simulink library "lib_outputs"  (Simulink 4.1.1)
undefined symbols (not defined in the file or in its folder): ess2_init_soc, ess_init_soc
libraries: lib_outputs x2
settings Model: LastModifiedBy=abrooker  ModifiedComment=abrooker -- Thu Apr 25 12:43:46 2002 -- Version 1.75
settings Model: ModifiedHistory=|
  | abrooker -- Thu Apr 25 12:43:46 2002 -- Version 1.75
  | 
  | 
  | abrooker -- Thu Apr 25 12:43:39 2002 -- Version 1.74
  | 
  | 
  | abrooker -- Thu Apr 25 12:37:48 2002 -- Version 1.73
  | 
  | 
  | abrooker -- Thu Apr 25 11:19:32 2002 -- Version 1.72
  | 
  | 
  | abrooker -- Thu Apr 25 11:09:29 2002 -- Version 1.71
  | 
  | 
  | abrooker -- Thu Apr 25 11:09:22 2002 -- Version 1.70
  | 
  | 
  | mokeefe -- Thu Apr 18 08:37:41 2002 -- Version 1.69
  | saving the model:
  | o "without the model browser open"
  | o with only top-level screen visible
  | o with "fit to view" enabled
  | o with "status bar" off and "toolbar" off
  | o with "prompt to update model history with each save" on

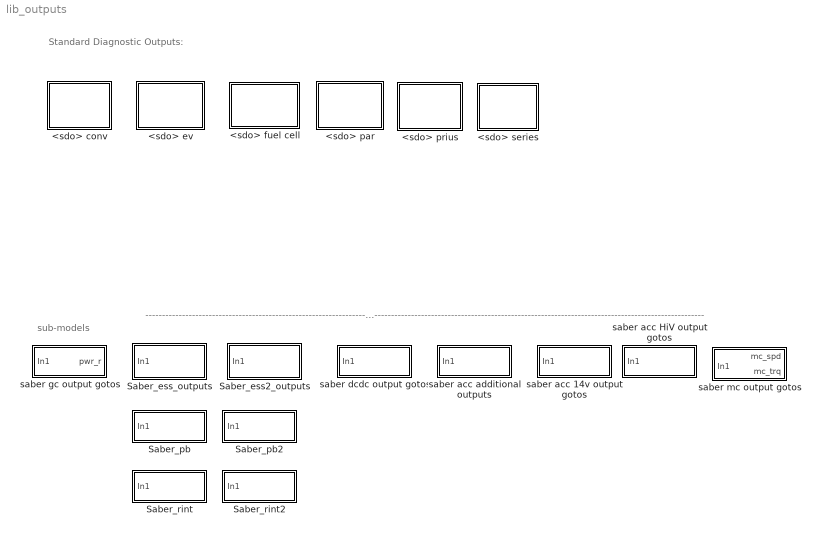
== system lib_outputs ==
  note: Standard Diagnostic Outputs:
  note: sub-models
  note: ------------------------------------------------------------------------------------------------------------------------------------------------------------------------------------------------------------------
  <sdo> conv : Subsystem
      settings: RTWFcnNameOpts=Auto  RTWFileNameOpts=Auto
      mask Display: image(imread('bdi_sdo.jpg'))
  <sdo> ev : Subsystem
      settings: RTWFcnNameOpts=Auto  RTWFileNameOpts=Auto
      mask Display: image(imread('bdi_sdo.jpg'))
  <sdo> fuel cell : Subsystem
      settings: RTWFcnNameOpts=Auto  RTWFileNameOpts=Auto
      mask Display: image(imread('bdi_sdo.jpg'))
  <sdo> par : Subsystem
      settings: RTWFcnNameOpts=Auto  RTWFileNameOpts=Auto
      mask Display: image(imread('bdi_sdo.jpg'))
  <sdo> prius : Subsystem
      settings: RTWFcnNameOpts=Auto  RTWFileNameOpts=Auto
      mask Display: image(imread('bdi_sdo.jpg'))
  <sdo> series : Subsystem
      settings: RTWFcnNameOpts=Auto  RTWFileNameOpts=Auto
      mask Display: image(imread('bdi_sdo.jpg'))
  Saber_ess2_outputs : Subsystem  BlockChoice=Saber_rint2
      settings: TemplateBlock=self  MemberBlocks=Saber_pb2,Saber_rint2  RTWFcnNameOpts=Auto  RTWFileNameOpts=Auto
  Saber_ess_outputs : Subsystem  BlockChoice=Saber_rint
      settings: TemplateBlock=self  MemberBlocks=Saber_pb,Saber_rint  RTWFcnNameOpts=Auto  RTWFileNameOpts=Auto
  Saber_pb : Subsystem
      settings: RTWFcnNameOpts=Auto  RTWFileNameOpts=Auto
  Saber_pb2 : Subsystem
      settings: RTWFcnNameOpts=Auto  RTWFileNameOpts=Auto
  Saber_rint : Subsystem
      settings: RTWFcnNameOpts=Auto  RTWFileNameOpts=Auto
  Saber_rint2 : Subsystem
      settings: RTWFcnNameOpts=Auto  RTWFileNameOpts=Auto
  saber acc 14v output gotos : Subsystem
      settings: RTWFcnNameOpts=Auto  RTWFileNameOpts=Auto
  saber acc HiV output gotos : Subsystem
      settings: RTWFcnNameOpts=Auto  RTWFileNameOpts=Auto
  saber acc additional outputs : Subsystem
      settings: RTWFcnNameOpts=Auto  RTWFileNameOpts=Auto
  saber dcdc output gotos : Subsystem
      settings: RTWFcnNameOpts=Auto  RTWFileNameOpts=Auto
  saber gc output gotos : Subsystem
      settings: RTWFcnNameOpts=Auto  RTWFileNameOpts=Auto
  saber mc output gotos : Subsystem
      settings: RTWFcnNameOpts=Auto  RTWFileNameOpts=Auto

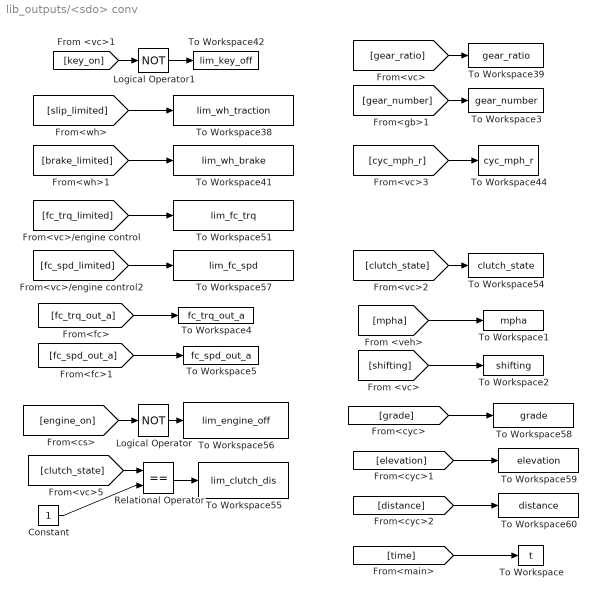
== system lib_outputs/<sdo> conv ==
  Constant : Constant  Value=1
  Logical Operator : Logic  Operator=NOT  Inputs=1
  Logical Operator1 : Logic  Operator=NOT  Inputs=1
  Relational Operator : RelationalOperator  Operator===
  To Workspace : ToWorkspace  VariableName=t  SampleTime=0  SaveFormat=Array
  To Workspace1 : ToWorkspace  VariableName=mpha  SampleTime=-1  SaveFormat=Array
  To Workspace2 : ToWorkspace  VariableName=shifting  SampleTime=-1  SaveFormat=Array
  To Workspace3 : ToWorkspace  VariableName=gear_number  SampleTime=-1  SaveFormat=Array
  To Workspace38 : ToWorkspace  VariableName=lim_wh_traction  SampleTime=-1  SaveFormat=Array
  To Workspace39 : ToWorkspace  VariableName=gear_ratio  SampleTime=-1  SaveFormat=Array
  To Workspace4 : ToWorkspace  VariableName=fc_trq_out_a  SampleTime=-1  SaveFormat=Array
  To Workspace41 : ToWorkspace  VariableName=lim_wh_brake  SampleTime=-1  SaveFormat=Array
  To Workspace42 : ToWorkspace  VariableName=lim_key_off  SampleTime=-1  SaveFormat=Array
  To Workspace44 : ToWorkspace  VariableName=cyc_mph_r  SampleTime=-1  SaveFormat=Array
  To Workspace5 : ToWorkspace  VariableName=fc_spd_out_a  SampleTime=-1  SaveFormat=Array
  To Workspace51 : ToWorkspace  VariableName=lim_fc_trq  SampleTime=-1  SaveFormat=Array
  To Workspace54 : ToWorkspace  VariableName=clutch_state  SampleTime=-1  SaveFormat=Array
  To Workspace55 : ToWorkspace  VariableName=lim_clutch_dis  SampleTime=-1  SaveFormat=Array
  To Workspace56 : ToWorkspace  VariableName=lim_engine_off  SampleTime=-1  SaveFormat=Array
  To Workspace57 : ToWorkspace  VariableName=lim_fc_spd  SampleTime=-1  SaveFormat=Array
  To Workspace58 : ToWorkspace  VariableName=grade  SampleTime=-1  SaveFormat=Array
  To Workspace59 : ToWorkspace  VariableName=elevation  SampleTime=-1  SaveFormat=Array
  To Workspace60 : ToWorkspace  VariableName=distance  SampleTime=-1  SaveFormat=Array
  wires:
  [gear_ratio] -> To Workspace39/1
  [cyc_mph_r] -> To Workspace44/1
  [clutch_state] -> To Workspace54/1
  [mpha] -> To Workspace1/1
  [shifting] -> To Workspace2/1
  [slip_limited] -> To Workspace38/1
  [brake_limited] -> To Workspace41/1
  [fc_trq_limited] -> To Workspace51/1
  [fc_spd_limited] -> To Workspace57/1
  [key_on] -> Logical Operator1/1
  Logical Operator1/1 -> To Workspace42/1
  [grade] -> To Workspace58/1
  [elevation] -> To Workspace59/1
  [distance] -> To Workspace60/1
  [clutch_state] -> Relational Operator/1
  Relational Operator/1 -> To Workspace55/1
  Constant/1 -> Relational Operator/2
  [engine_on] -> Logical Operator/1
  Logical Operator/1 -> To Workspace56/1
  [fc_trq_out_a] -> To Workspace4/1
  [fc_spd_out_a] -> To Workspace5/1
  [time] -> To Workspace/1
  [gear_number] -> To Workspace3/1

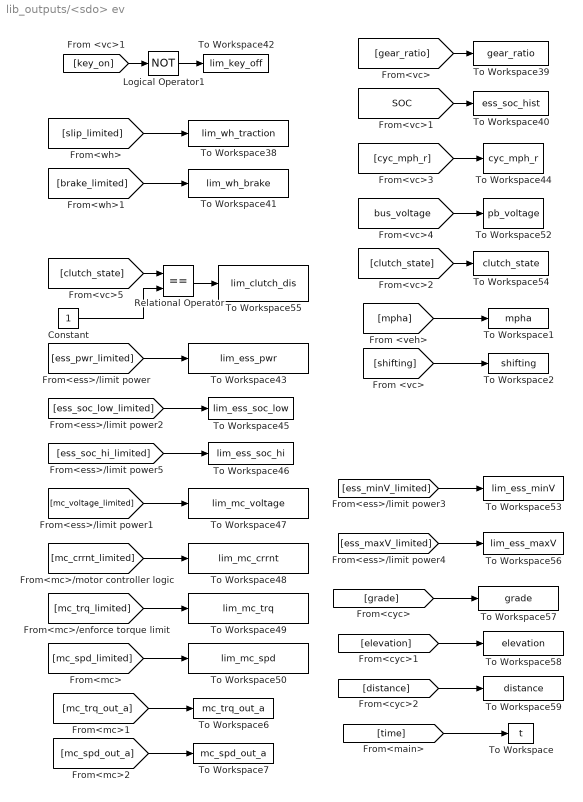
== system lib_outputs/<sdo> ev ==
  Constant : Constant  Value=1
  Logical Operator1 : Logic  Operator=NOT  Inputs=1
  Relational Operator : RelationalOperator  Operator===
  To Workspace : ToWorkspace  VariableName=t  SampleTime=0  SaveFormat=Array
  To Workspace1 : ToWorkspace  VariableName=mpha  SampleTime=-1  SaveFormat=Array
  To Workspace2 : ToWorkspace  VariableName=shifting  SampleTime=-1  SaveFormat=Array
  To Workspace38 : ToWorkspace  VariableName=lim_wh_traction  SampleTime=-1  SaveFormat=Array
  To Workspace39 : ToWorkspace  VariableName=gear_ratio  SampleTime=-1  SaveFormat=Array
  To Workspace40 : ToWorkspace  VariableName=ess_soc_hist  SampleTime=-1  SaveFormat=Array
  To Workspace41 : ToWorkspace  VariableName=lim_wh_brake  SampleTime=-1  SaveFormat=Array
  To Workspace42 : ToWorkspace  VariableName=lim_key_off  SampleTime=-1  SaveFormat=Array
  To Workspace43 : ToWorkspace  VariableName=lim_ess_pwr  SampleTime=-1  SaveFormat=Array
  To Workspace44 : ToWorkspace  VariableName=cyc_mph_r  SampleTime=-1  SaveFormat=Array
  To Workspace45 : ToWorkspace  VariableName=lim_ess_soc_low  SampleTime=-1  SaveFormat=Array
  To Workspace46 : ToWorkspace  VariableName=lim_ess_soc_hi  SampleTime=-1  SaveFormat=Array
  To Workspace47 : ToWorkspace  VariableName=lim_mc_voltage  SampleTime=-1  SaveFormat=Array
  To Workspace48 : ToWorkspace  VariableName=lim_mc_crrnt  SampleTime=-1  SaveFormat=Array
  To Workspace49 : ToWorkspace  VariableName=lim_mc_trq  SampleTime=-1  SaveFormat=Array
  To Workspace50 : ToWorkspace  VariableName=lim_mc_spd  SampleTime=-1  SaveFormat=Array
  To Workspace52 : ToWorkspace  VariableName=pb_voltage  SampleTime=-1  SaveFormat=Array
  To Workspace53 : ToWorkspace  VariableName=lim_ess_minV  SampleTime=-1  SaveFormat=Array
  To Workspace54 : ToWorkspace  VariableName=clutch_state  SampleTime=-1  SaveFormat=Array
  To Workspace55 : ToWorkspace  VariableName=lim_clutch_dis  SampleTime=-1  SaveFormat=Array
  To Workspace56 : ToWorkspace  VariableName=lim_ess_maxV  SampleTime=-1  SaveFormat=Array
  To Workspace57 : ToWorkspace  VariableName=grade  SampleTime=-1  SaveFormat=Array
  To Workspace58 : ToWorkspace  VariableName=elevation  SampleTime=-1  SaveFormat=Array
  To Workspace59 : ToWorkspace  VariableName=distance  SampleTime=-1  SaveFormat=Array
  To Workspace6 : ToWorkspace  VariableName=mc_trq_out_a  SampleTime=-1  SaveFormat=Array
  To Workspace7 : ToWorkspace  VariableName=mc_spd_out_a  SampleTime=-1  SaveFormat=Array
  wires:
  [mc_voltage_limited] -> To Workspace47/1
  [mc_crrnt_limited] -> To Workspace48/1
  [mc_trq_limited] -> To Workspace49/1
  [mc_spd_limited] -> To Workspace50/1
  [gear_ratio] -> To Workspace39/1
  [cyc_mph_r] -> To Workspace44/1
  [SOC] -> To Workspace40/1
  [bus_voltage] -> To Workspace52/1
  [clutch_state] -> To Workspace54/1
  [mpha] -> To Workspace1/1
  [shifting] -> To Workspace2/1
  [slip_limited] -> To Workspace38/1
  [brake_limited] -> To Workspace41/1
  [key_on] -> Logical Operator1/1
  Logical Operator1/1 -> To Workspace42/1
  [ess_maxV_limited] -> To Workspace56/1
  [ess_minV_limited] -> To Workspace53/1
  [grade] -> To Workspace57/1
  [elevation] -> To Workspace58/1
  [distance] -> To Workspace59/1
  [ess_pwr_limited] -> To Workspace43/1
  [clutch_state] -> Relational Operator/1
  Relational Operator/1 -> To Workspace55/1
  Constant/1 -> Relational Operator/2
  [ess_soc_low_limited] -> To Workspace45/1
  [ess_soc_hi_limited] -> To Workspace46/1
  [time] -> To Workspace/1
  [mc_trq_out_a] -> To Workspace6/1
  [mc_spd_out_a] -> To Workspace7/1

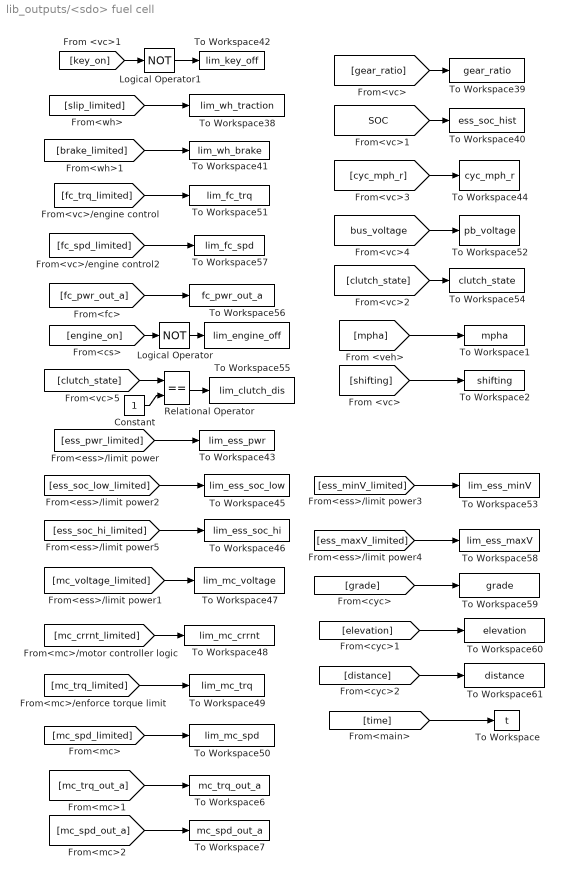
== system lib_outputs/<sdo> fuel cell ==
  " " : ToWorkspace  VariableName=fc_pwr_out_a  SampleTime=-1  SaveFormat=Array
  Constant : Constant  Value=1
  Logical Operator : Logic  Operator=NOT  Inputs=1
  Logical Operator1 : Logic  Operator=NOT  Inputs=1
  Relational Operator : RelationalOperator  Operator===
  To Workspace : ToWorkspace  VariableName=t  SampleTime=0  SaveFormat=Array
  To Workspace1 : ToWorkspace  VariableName=mpha  SampleTime=-1  SaveFormat=Array
  To Workspace2 : ToWorkspace  VariableName=shifting  SampleTime=-1  SaveFormat=Array
  To Workspace38 : ToWorkspace  VariableName=lim_wh_traction  SampleTime=-1  SaveFormat=Array
  To Workspace39 : ToWorkspace  VariableName=gear_ratio  SampleTime=-1  SaveFormat=Array
  To Workspace40 : ToWorkspace  VariableName=ess_soc_hist  SampleTime=-1  SaveFormat=Array
  To Workspace41 : ToWorkspace  VariableName=lim_wh_brake  SampleTime=-1  SaveFormat=Array
  To Workspace42 : ToWorkspace  VariableName=lim_key_off  SampleTime=-1  SaveFormat=Array
  To Workspace43 : ToWorkspace  VariableName=lim_ess_pwr  SampleTime=-1  SaveFormat=Array
  To Workspace44 : ToWorkspace  VariableName=cyc_mph_r  SampleTime=-1  SaveFormat=Array
  To Workspace45 : ToWorkspace  VariableName=lim_ess_soc_low  SampleTime=-1  SaveFormat=Array
  To Workspace46 : ToWorkspace  VariableName=lim_ess_soc_hi  SampleTime=-1  SaveFormat=Array
  To Workspace47 : ToWorkspace  VariableName=lim_mc_voltage  SampleTime=-1  SaveFormat=Array
  To Workspace48 : ToWorkspace  VariableName=lim_mc_crrnt  SampleTime=-1  SaveFormat=Array
  To Workspace49 : ToWorkspace  VariableName=lim_mc_trq  SampleTime=-1  SaveFormat=Array
  To Workspace50 : ToWorkspace  VariableName=lim_mc_spd  SampleTime=-1  SaveFormat=Array
  To Workspace51 : ToWorkspace  VariableName=lim_fc_trq  SampleTime=-1  SaveFormat=Array
  To Workspace52 : ToWorkspace  VariableName=pb_voltage  SampleTime=-1  SaveFormat=Array
  To Workspace53 : ToWorkspace  VariableName=lim_ess_minV  SampleTime=-1  SaveFormat=Array
  To Workspace54 : ToWorkspace  VariableName=clutch_state  SampleTime=-1  SaveFormat=Array
  To Workspace55 : ToWorkspace  VariableName=lim_clutch_dis  SampleTime=-1  SaveFormat=Array
  To Workspace56 : ToWorkspace  VariableName=lim_engine_off  SampleTime=-1  SaveFormat=Array
  To Workspace57 : ToWorkspace  VariableName=lim_fc_spd  SampleTime=-1  SaveFormat=Array
  To Workspace58 : ToWorkspace  VariableName=lim_ess_maxV  SampleTime=-1  SaveFormat=Array
  To Workspace59 : ToWorkspace  VariableName=grade  SampleTime=-1  SaveFormat=Array
  To Workspace6 : ToWorkspace  VariableName=mc_trq_out_a  SampleTime=-1  SaveFormat=Array
  To Workspace60 : ToWorkspace  VariableName=elevation  SampleTime=-1  SaveFormat=Array
  To Workspace61 : ToWorkspace  VariableName=distance  SampleTime=-1  SaveFormat=Array
  To Workspace7 : ToWorkspace  VariableName=mc_spd_out_a  SampleTime=-1  SaveFormat=Array
  wires:
  [fc_trq_limited] -> To Workspace51/1
  [fc_spd_limited] -> To Workspace57/1
  [brake_limited] -> To Workspace41/1
  [slip_limited] -> To Workspace38/1
  [gear_ratio] -> To Workspace39/1
  [cyc_mph_r] -> To Workspace44/1
  [SOC] -> To Workspace40/1
  [bus_voltage] -> To Workspace52/1
  [clutch_state] -> To Workspace54/1
  [mpha] -> To Workspace1/1
  [shifting] -> To Workspace2/1
  [key_on] -> Logical Operator1/1
  Logical Operator1/1 -> To Workspace42/1
  [ess_maxV_limited] -> To Workspace58/1
  [ess_minV_limited] -> To Workspace53/1
  [grade] -> To Workspace59/1
  [elevation] -> To Workspace60/1
  [distance] -> To Workspace61/1
  [clutch_state] -> Relational Operator/1
  Relational Operator/1 -> To Workspace55/1
  Constant/1 -> Relational Operator/2
  [engine_on] -> Logical Operator/1
  Logical Operator/1 -> To Workspace56/1
  [ess_pwr_limited] -> To Workspace43/1
  [mc_voltage_limited] -> To Workspace47/1
  [mc_crrnt_limited] -> To Workspace48/1
  [mc_trq_limited] -> To Workspace49/1
  [mc_spd_limited] -> To Workspace50/1
  [ess_soc_low_limited] -> To Workspace45/1
  [ess_soc_hi_limited] -> To Workspace46/1
  [fc_pwr_out_a] -> " "/1
  [time] -> To Workspace/1
  [mc_trq_out_a] -> To Workspace6/1
  [mc_spd_out_a] -> To Workspace7/1

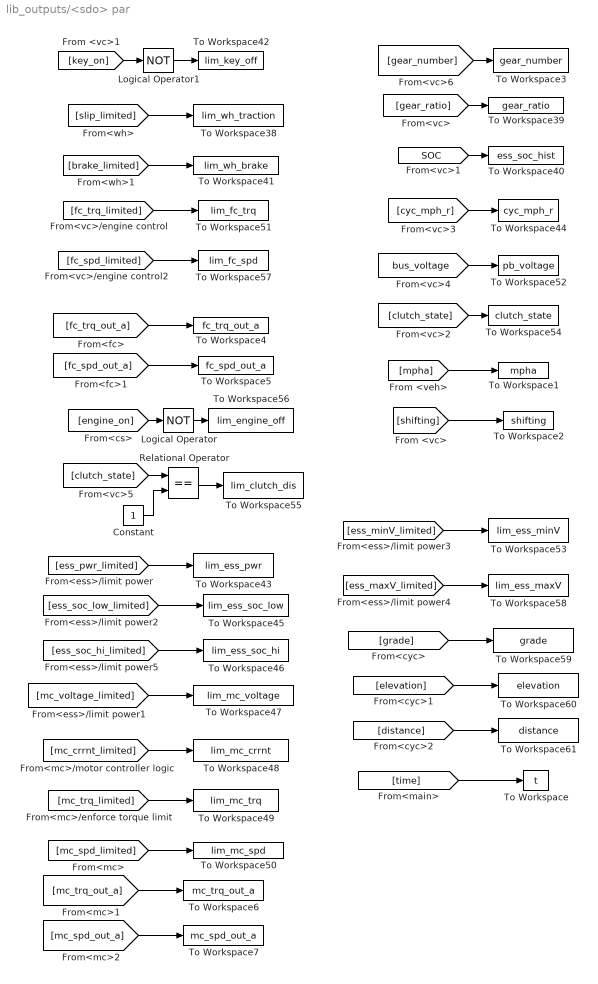
== system lib_outputs/<sdo> par ==
  Constant : Constant  Value=1
  Logical Operator : Logic  Operator=NOT  Inputs=1
  Logical Operator1 : Logic  Operator=NOT  Inputs=1
  Relational Operator : RelationalOperator  Operator===
  To Workspace : ToWorkspace  VariableName=t  SampleTime=0  SaveFormat=Array
  To Workspace1 : ToWorkspace  VariableName=mpha  SampleTime=-1  SaveFormat=Array
  To Workspace2 : ToWorkspace  VariableName=shifting  SampleTime=-1  SaveFormat=Array
  To Workspace3 : ToWorkspace  VariableName=gear_number  SampleTime=-1  SaveFormat=Array
  To Workspace38 : ToWorkspace  VariableName=lim_wh_traction  SampleTime=-1  SaveFormat=Array
  To Workspace39 : ToWorkspace  VariableName=gear_ratio  SampleTime=-1  SaveFormat=Array
  To Workspace4 : ToWorkspace  VariableName=fc_trq_out_a  SampleTime=-1  SaveFormat=Array
  To Workspace40 : ToWorkspace  VariableName=ess_soc_hist  SampleTime=-1  SaveFormat=Array
  To Workspace41 : ToWorkspace  VariableName=lim_wh_brake  SampleTime=-1  SaveFormat=Array
  To Workspace42 : ToWorkspace  VariableName=lim_key_off  SampleTime=-1  SaveFormat=Array
  To Workspace43 : ToWorkspace  VariableName=lim_ess_pwr  SampleTime=-1  SaveFormat=Array
  To Workspace44 : ToWorkspace  VariableName=cyc_mph_r  SampleTime=-1  SaveFormat=Array
  To Workspace45 : ToWorkspace  VariableName=lim_ess_soc_low  SampleTime=-1  SaveFormat=Array
  To Workspace46 : ToWorkspace  VariableName=lim_ess_soc_hi  SampleTime=-1  SaveFormat=Array
  To Workspace47 : ToWorkspace  VariableName=lim_mc_voltage  SampleTime=-1  SaveFormat=Array
  To Workspace48 : ToWorkspace  VariableName=lim_mc_crrnt  SampleTime=-1  SaveFormat=Array
  To Workspace49 : ToWorkspace  VariableName=lim_mc_trq  SampleTime=-1  SaveFormat=Array
  To Workspace5 : ToWorkspace  VariableName=fc_spd_out_a  SampleTime=-1  SaveFormat=Array
  To Workspace50 : ToWorkspace  VariableName=lim_mc_spd  SampleTime=-1  SaveFormat=Array
  To Workspace51 : ToWorkspace  VariableName=lim_fc_trq  SampleTime=-1  SaveFormat=Array
  To Workspace52 : ToWorkspace  VariableName=pb_voltage  SampleTime=-1  SaveFormat=Array
  To Workspace53 : ToWorkspace  VariableName=lim_ess_minV  SampleTime=-1  SaveFormat=Array
  To Workspace54 : ToWorkspace  VariableName=clutch_state  SampleTime=-1  SaveFormat=Array
  To Workspace55 : ToWorkspace  VariableName=lim_clutch_dis  SampleTime=-1  SaveFormat=Array
  To Workspace56 : ToWorkspace  VariableName=lim_engine_off  SampleTime=-1  SaveFormat=Array
  To Workspace57 : ToWorkspace  VariableName=lim_fc_spd  SampleTime=-1  SaveFormat=Array
  To Workspace58 : ToWorkspace  VariableName=lim_ess_maxV  SampleTime=-1  SaveFormat=Array
  To Workspace59 : ToWorkspace  VariableName=grade  SampleTime=-1  SaveFormat=Array
  To Workspace6 : ToWorkspace  VariableName=mc_trq_out_a  SampleTime=-1  SaveFormat=Array
  To Workspace60 : ToWorkspace  VariableName=elevation  SampleTime=-1  SaveFormat=Array
  To Workspace61 : ToWorkspace  VariableName=distance  SampleTime=-1  SaveFormat=Array
  To Workspace7 : ToWorkspace  VariableName=mc_spd_out_a  SampleTime=-1  SaveFormat=Array
  wires:
  [fc_trq_limited] -> To Workspace51/1
  [fc_spd_limited] -> To Workspace57/1
  [gear_ratio] -> To Workspace39/1
  [cyc_mph_r] -> To Workspace44/1
  [SOC] -> To Workspace40/1
  [bus_voltage] -> To Workspace52/1
  [clutch_state] -> To Workspace54/1
  [mpha] -> To Workspace1/1
  [shifting] -> To Workspace2/1
  [key_on] -> Logical Operator1/1
  Logical Operator1/1 -> To Workspace42/1
  [slip_limited] -> To Workspace38/1
  [brake_limited] -> To Workspace41/1
  [ess_maxV_limited] -> To Workspace58/1
  [ess_minV_limited] -> To Workspace53/1
  [grade] -> To Workspace59/1
  [elevation] -> To Workspace60/1
  [distance] -> To Workspace61/1
  [ess_pwr_limited] -> To Workspace43/1
  [clutch_state] -> Relational Operator/1
  Constant/1 -> Relational Operator/2
  [engine_on] -> Logical Operator/1
  Logical Operator/1 -> To Workspace56/1
  [ess_soc_low_limited] -> To Workspace45/1
  [ess_soc_hi_limited] -> To Workspace46/1
  [mc_voltage_limited] -> To Workspace47/1
  [mc_crrnt_limited] -> To Workspace48/1
  [mc_trq_limited] -> To Workspace49/1
  [mc_spd_limited] -> To Workspace50/1
  Relational Operator/1 -> To Workspace55/1
  [fc_trq_out_a] -> To Workspace4/1
  [fc_spd_out_a] -> To Workspace5/1
  [time] -> To Workspace/1
  [mc_trq_out_a] -> To Workspace6/1
  [mc_spd_out_a] -> To Workspace7/1
  [gear_number] -> To Workspace3/1

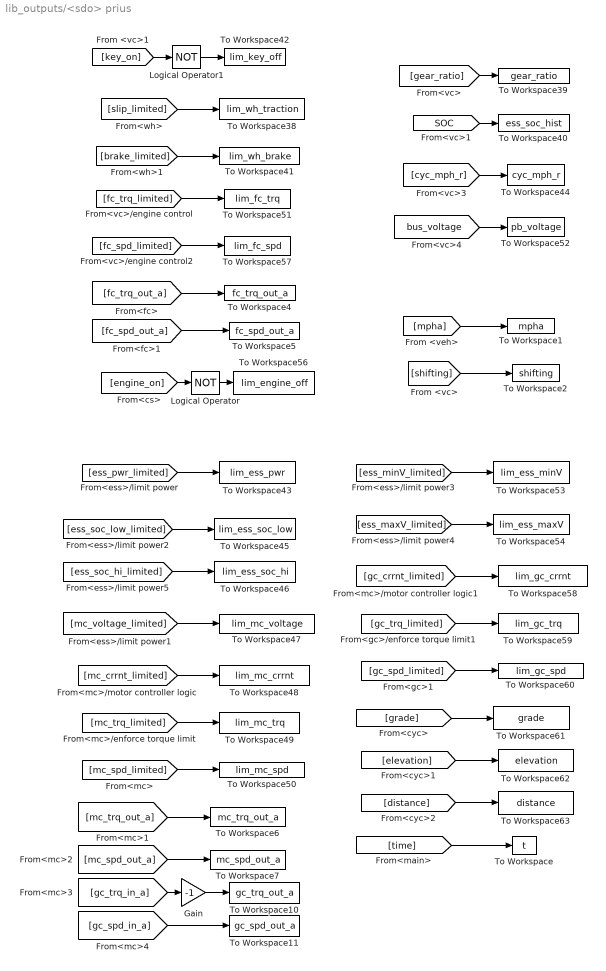
== system lib_outputs/<sdo> prius ==
  Gain : Gain  Gain=-1  Multiplication=Element-wise(K.*u)  SaturateOnIntegerOverflow=on
  Logical Operator : Logic  Operator=NOT  Inputs=1
  Logical Operator1 : Logic  Operator=NOT  Inputs=1
  To Workspace : ToWorkspace  VariableName=t  SampleTime=0  SaveFormat=Array
  To Workspace1 : ToWorkspace  VariableName=mpha  SampleTime=-1  SaveFormat=Array
  To Workspace10 : ToWorkspace  VariableName=gc_trq_out_a  SampleTime=-1  SaveFormat=Array
  To Workspace11 : ToWorkspace  VariableName=gc_spd_out_a  SampleTime=-1  SaveFormat=Array
  To Workspace2 : ToWorkspace  VariableName=shifting  SampleTime=-1  SaveFormat=Array
  To Workspace38 : ToWorkspace  VariableName=lim_wh_traction  SampleTime=-1  SaveFormat=Array
  To Workspace39 : ToWorkspace  VariableName=gear_ratio  SampleTime=-1  SaveFormat=Array
  To Workspace4 : ToWorkspace  VariableName=fc_trq_out_a  SampleTime=-1  SaveFormat=Array
  To Workspace40 : ToWorkspace  VariableName=ess_soc_hist  SampleTime=-1  SaveFormat=Array
  To Workspace41 : ToWorkspace  VariableName=lim_wh_brake  SampleTime=-1  SaveFormat=Array
  To Workspace42 : ToWorkspace  VariableName=lim_key_off  SampleTime=-1  SaveFormat=Array
  To Workspace43 : ToWorkspace  VariableName=lim_ess_pwr  SampleTime=-1  SaveFormat=Array
  To Workspace44 : ToWorkspace  VariableName=cyc_mph_r  SampleTime=-1  SaveFormat=Array
  To Workspace45 : ToWorkspace  VariableName=lim_ess_soc_low  SampleTime=-1  SaveFormat=Array
  To Workspace46 : ToWorkspace  VariableName=lim_ess_soc_hi  SampleTime=-1  SaveFormat=Array
  To Workspace47 : ToWorkspace  VariableName=lim_mc_voltage  SampleTime=-1  SaveFormat=Array
  To Workspace48 : ToWorkspace  VariableName=lim_mc_crrnt  SampleTime=-1  SaveFormat=Array
  To Workspace49 : ToWorkspace  VariableName=lim_mc_trq  SampleTime=-1  SaveFormat=Array
  To Workspace5 : ToWorkspace  VariableName=fc_spd_out_a  SampleTime=-1  SaveFormat=Array
  To Workspace50 : ToWorkspace  VariableName=lim_mc_spd  SampleTime=-1  SaveFormat=Array
  To Workspace51 : ToWorkspace  VariableName=lim_fc_trq  SampleTime=-1  SaveFormat=Array
  To Workspace52 : ToWorkspace  VariableName=pb_voltage  SampleTime=-1  SaveFormat=Array
  To Workspace53 : ToWorkspace  VariableName=lim_ess_minV  SampleTime=-1  SaveFormat=Array
  To Workspace54 : ToWorkspace  VariableName=lim_ess_maxV  SampleTime=-1  SaveFormat=Array
  To Workspace56 : ToWorkspace  VariableName=lim_engine_off  SampleTime=-1  SaveFormat=Array
  To Workspace57 : ToWorkspace  VariableName=lim_fc_spd  SampleTime=-1  SaveFormat=Array
  To Workspace58 : ToWorkspace  VariableName=lim_gc_crrnt  SampleTime=-1  SaveFormat=Array
  To Workspace59 : ToWorkspace  VariableName=lim_gc_trq  SampleTime=-1  SaveFormat=Array
  To Workspace6 : ToWorkspace  VariableName=mc_trq_out_a  SampleTime=-1  SaveFormat=Array
  To Workspace60 : ToWorkspace  VariableName=lim_gc_spd  SampleTime=-1  SaveFormat=Array
  To Workspace61 : ToWorkspace  VariableName=grade  SampleTime=-1  SaveFormat=Array
  To Workspace62 : ToWorkspace  VariableName=elevation  SampleTime=-1  SaveFormat=Array
  To Workspace63 : ToWorkspace  VariableName=distance  SampleTime=-1  SaveFormat=Array
  To Workspace7 : ToWorkspace  VariableName=mc_spd_out_a  SampleTime=-1  SaveFormat=Array
  wires:
  [distance] -> To Workspace63/1
  [elevation] -> To Workspace62/1
  [grade] -> To Workspace61/1
  [gc_spd_limited] -> To Workspace60/1
  [gc_trq_limited] -> To Workspace59/1
  [gc_crrnt_limited] -> To Workspace58/1
  [ess_minV_limited] -> To Workspace53/1
  [ess_maxV_limited] -> To Workspace54/1
  [brake_limited] -> To Workspace41/1
  [slip_limited] -> To Workspace38/1
  Logical Operator1/1 -> To Workspace42/1
  [key_on] -> Logical Operator1/1
  [shifting] -> To Workspace2/1
  [mpha] -> To Workspace1/1
  [bus_voltage] -> To Workspace52/1
  [SOC] -> To Workspace40/1
  [cyc_mph_r] -> To Workspace44/1
  [gear_ratio] -> To Workspace39/1
  [fc_spd_limited] -> To Workspace57/1
  [fc_trq_limited] -> To Workspace51/1
  [ess_soc_hi_limited] -> To Workspace46/1
  [ess_soc_low_limited] -> To Workspace45/1
  [ess_pwr_limited] -> To Workspace43/1
  Logical Operator/1 -> To Workspace56/1
  [engine_on] -> Logical Operator/1
  [mc_spd_limited] -> To Workspace50/1
  [mc_trq_limited] -> To Workspace49/1
  [mc_crrnt_limited] -> To Workspace48/1
  [mc_voltage_limited] -> To Workspace47/1
  [fc_trq_out_a] -> To Workspace4/1
  [fc_spd_out_a] -> To Workspace5/1
  [time] -> To Workspace/1
  [mc_trq_out_a] -> To Workspace6/1
  [mc_spd_out_a] -> To Workspace7/1
  [gc_trq_in_a] -> Gain/1
  Gain/1 -> To Workspace10/1
  [gc_spd_in_a] -> To Workspace11/1

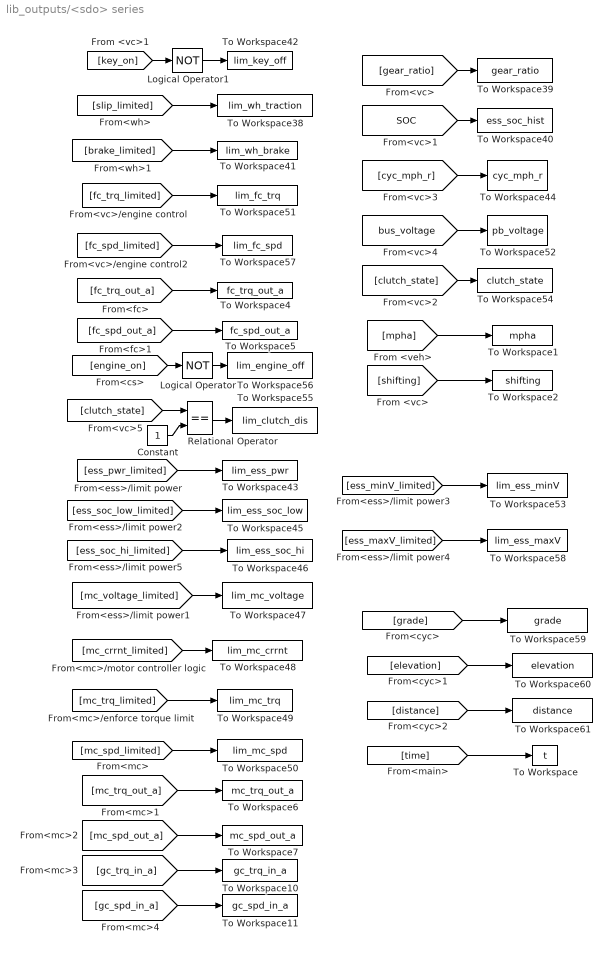
== system lib_outputs/<sdo> series ==
  Constant : Constant  Value=1
  Logical Operator : Logic  Operator=NOT  Inputs=1
  Logical Operator1 : Logic  Operator=NOT  Inputs=1
  Relational Operator : RelationalOperator  Operator===
  To Workspace : ToWorkspace  VariableName=t  SampleTime=0  SaveFormat=Array
  To Workspace1 : ToWorkspace  VariableName=mpha  SampleTime=-1  SaveFormat=Array
  To Workspace10 : ToWorkspace  VariableName=gc_trq_in_a  SampleTime=-1  SaveFormat=Array
  To Workspace11 : ToWorkspace  VariableName=gc_spd_in_a  SampleTime=-1  SaveFormat=Array
  To Workspace2 : ToWorkspace  VariableName=shifting  SampleTime=-1  SaveFormat=Array
  To Workspace38 : ToWorkspace  VariableName=lim_wh_traction  SampleTime=-1  SaveFormat=Array
  To Workspace39 : ToWorkspace  VariableName=gear_ratio  SampleTime=-1  SaveFormat=Array
  To Workspace4 : ToWorkspace  VariableName=fc_trq_out_a  SampleTime=-1  SaveFormat=Array
  To Workspace40 : ToWorkspace  VariableName=ess_soc_hist  SampleTime=-1  SaveFormat=Array
  To Workspace41 : ToWorkspace  VariableName=lim_wh_brake  SampleTime=-1  SaveFormat=Array
  To Workspace42 : ToWorkspace  VariableName=lim_key_off  SampleTime=-1  SaveFormat=Array
  To Workspace43 : ToWorkspace  VariableName=lim_ess_pwr  SampleTime=-1  SaveFormat=Array
  To Workspace44 : ToWorkspace  VariableName=cyc_mph_r  SampleTime=-1  SaveFormat=Array
  To Workspace45 : ToWorkspace  VariableName=lim_ess_soc_low  SampleTime=-1  SaveFormat=Array
  To Workspace46 : ToWorkspace  VariableName=lim_ess_soc_hi  SampleTime=-1  SaveFormat=Array
  To Workspace47 : ToWorkspace  VariableName=lim_mc_voltage  SampleTime=-1  SaveFormat=Array
  To Workspace48 : ToWorkspace  VariableName=lim_mc_crrnt  SampleTime=-1  SaveFormat=Array
  To Workspace49 : ToWorkspace  VariableName=lim_mc_trq  SampleTime=-1  SaveFormat=Array
  To Workspace5 : ToWorkspace  VariableName=fc_spd_out_a  SampleTime=-1  SaveFormat=Array
  To Workspace50 : ToWorkspace  VariableName=lim_mc_spd  SampleTime=-1  SaveFormat=Array
  To Workspace51 : ToWorkspace  VariableName=lim_fc_trq  SampleTime=-1  SaveFormat=Array
  To Workspace52 : ToWorkspace  VariableName=pb_voltage  SampleTime=-1  SaveFormat=Array
  To Workspace53 : ToWorkspace  VariableName=lim_ess_minV  SampleTime=-1  SaveFormat=Array
  To Workspace54 : ToWorkspace  VariableName=clutch_state  SampleTime=-1  SaveFormat=Array
  To Workspace55 : ToWorkspace  VariableName=lim_clutch_dis  SampleTime=-1  SaveFormat=Array
  To Workspace56 : ToWorkspace  VariableName=lim_engine_off  SampleTime=-1  SaveFormat=Array
  To Workspace57 : ToWorkspace  VariableName=lim_fc_spd  SampleTime=-1  SaveFormat=Array
  To Workspace58 : ToWorkspace  VariableName=lim_ess_maxV  SampleTime=-1  SaveFormat=Array
  To Workspace59 : ToWorkspace  VariableName=grade  SampleTime=-1  SaveFormat=Array
  To Workspace6 : ToWorkspace  VariableName=mc_trq_out_a  SampleTime=-1  SaveFormat=Array
  To Workspace60 : ToWorkspace  VariableName=elevation  SampleTime=-1  SaveFormat=Array
  To Workspace61 : ToWorkspace  VariableName=distance  SampleTime=-1  SaveFormat=Array
  To Workspace7 : ToWorkspace  VariableName=mc_spd_out_a  SampleTime=-1  SaveFormat=Array
  wires:
  [fc_trq_limited] -> To Workspace51/1
  [fc_spd_limited] -> To Workspace57/1
  [brake_limited] -> To Workspace41/1
  [slip_limited] -> To Workspace38/1
  [gear_ratio] -> To Workspace39/1
  [cyc_mph_r] -> To Workspace44/1
  [SOC] -> To Workspace40/1
  [bus_voltage] -> To Workspace52/1
  [clutch_state] -> To Workspace54/1
  [mpha] -> To Workspace1/1
  [shifting] -> To Workspace2/1
  [key_on] -> Logical Operator1/1
  Logical Operator1/1 -> To Workspace42/1
  [ess_maxV_limited] -> To Workspace58/1
  [ess_minV_limited] -> To Workspace53/1
  [grade] -> To Workspace59/1
  [elevation] -> To Workspace60/1
  [distance] -> To Workspace61/1
  Relational Operator/1 -> To Workspace55/1
  Constant/1 -> Relational Operator/2
  [engine_on] -> Logical Operator/1
  Logical Operator/1 -> To Workspace56/1
  [ess_pwr_limited] -> To Workspace43/1
  [ess_soc_low_limited] -> To Workspace45/1
  [ess_soc_hi_limited] -> To Workspace46/1
  [mc_voltage_limited] -> To Workspace47/1
  [mc_crrnt_limited] -> To Workspace48/1
  [mc_trq_limited] -> To Workspace49/1
  [mc_spd_limited] -> To Workspace50/1
  [fc_trq_out_a] -> To Workspace4/1
  [fc_spd_out_a] -> To Workspace5/1
  [clutch_state] -> Relational Operator/1
  [time] -> To Workspace/1
  [mc_trq_out_a] -> To Workspace6/1
  [mc_spd_out_a] -> To Workspace7/1
  [gc_trq_in_a] -> To Workspace10/1
  [gc_spd_in_a] -> To Workspace11/1

== system lib_outputs/Saber_ess2_outputs ==
  In1 : Inport  Port=1  LatchInput=off
  Saber_rint2 : lib_outputs/Saber_rint2
      settings: RTWFcnNameOpts=Auto  RTWFileNameOpts=Auto
  wires:
  In1/1 -> Saber_rint2/1

== system lib_outputs/Saber_ess_outputs ==
  In1 : Inport  Port=1  LatchInput=off
  Saber_rint : lib_outputs/Saber_rint
      settings: RTWFcnNameOpts=Auto  RTWFileNameOpts=Auto
  wires:
  In1/1 -> Saber_rint/1

== system lib_outputs/Saber_pb ==
  In1 : Inport  Port=1  LatchInput=off
  Advisor sign convention1 : Gain  Gain=-1  Multiplication=Element-wise(K.*u)  SaturateOnIntegerOverflow=on
  Demux : Demux  Outputs=4  BusSelectionMode=off
  Memory : Memory  X0=ess_init_soc  InheritSampleTime=off
      settings: RTWStateStorageClass=Auto
  Memory2 : Memory  X0=0  InheritSampleTime=off
      settings: RTWStateStorageClass=Auto
  Product : Product  Inputs=*/  Multiplication=Element-wise(.*)  SaturateOnIntegerOverflow=on
  Terminator : Terminator
  To Workspace1 : ToWorkspace  VariableName=ess_current  SampleTime=-1  SaveFormat=Array
  To Workspace2 : ToWorkspace  VariableName=ess_volts  SampleTime=-1  SaveFormat=Array
  To Workspace3 : ToWorkspace  VariableName=ess_current_psc  SampleTime=-1  SaveFormat=Array
  To Workspace4 : ToWorkspace  VariableName=ess_soc_hist  SampleTime=-1  SaveFormat=Array
  To Workspace5 : ToWorkspace  VariableName=ess_pwr_out_a  SampleTime=-1  SaveFormat=Array
  psc passive sign convention : Gain  Gain=-1  Multiplication=Element-wise(K.*u)  SaturateOnIntegerOverflow=on
  tag scope: SOC=global, bus_voltage=global, ess_pwr_out_a=global
  wires:
  Demux/3 -> To Workspace4/1, Memory/1
  In1/1 -> Demux/1
  Demux/1 -> Advisor sign convention1/1
  Demux/2 -> To Workspace2/1, Product/2, Memory2/1
  Product/1 -> To Workspace1/1, psc passive sign convention/1
  Memory/1 -> [SOC]
  Memory2/1 -> [bus_voltage]
  Demux/4 -> Terminator/1
  psc passive sign convention/1 -> To Workspace3/1
  Advisor sign convention1/1 -> To Workspace5/1, Product/1, [ess_pwr_out_a]

== system lib_outputs/Saber_pb2 ==
  In1 : Inport  Port=1  LatchInput=off
  Advisor sign convention1 : Gain  Gain=-1  Multiplication=Element-wise(K.*u)  SaturateOnIntegerOverflow=on
  Demux : Demux  Outputs=4  BusSelectionMode=off
  Product : Product  Inputs=*/  Multiplication=Element-wise(.*)  SaturateOnIntegerOverflow=on
  Terminator : Terminator
  To Workspace1 : ToWorkspace  VariableName=ess2_current  SampleTime=-1  SaveFormat=Array
  To Workspace2 : ToWorkspace  VariableName=ess2_volts  SampleTime=-1  SaveFormat=Array
  To Workspace3 : ToWorkspace  VariableName=ess2_current_psc  SampleTime=-1  SaveFormat=Array
  To Workspace4 : ToWorkspace  VariableName=ess2_soc_hist  SampleTime=-1  SaveFormat=Array
  To Workspace5 : ToWorkspace  VariableName=ess2_pwr_out_a  SampleTime=-1  SaveFormat=Array
  psc passive sign convention : Gain  Gain=-1  Multiplication=Element-wise(K.*u)  SaturateOnIntegerOverflow=on
  tag scope: ess2_pwr_out_a=global
  wires:
  Product/1 -> To Workspace1/1, psc passive sign convention/1
  Demux/2 -> Product/2, To Workspace2/1
  Demux/1 -> Advisor sign convention1/1
  In1/1 -> Demux/1
  Demux/3 -> To Workspace4/1
  Demux/4 -> Terminator/1
  psc passive sign convention/1 -> To Workspace3/1
  Advisor sign convention1/1 -> Product/1, To Workspace5/1, [ess2_pwr_out_a]

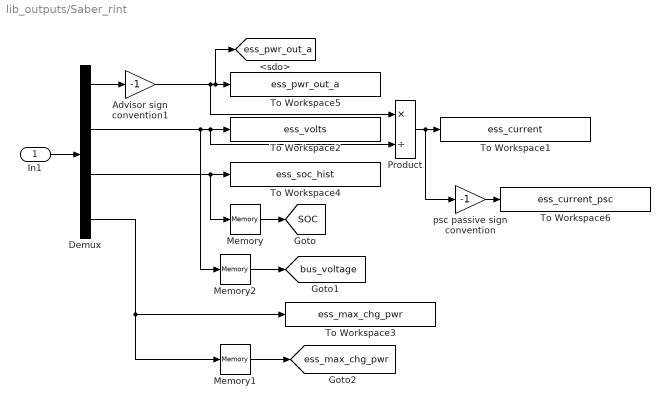
== system lib_outputs/Saber_rint ==
  In1 : Inport  Port=1  LatchInput=off
  Advisor sign convention1 : Gain  Gain=-1  Multiplication=Element-wise(K.*u)  SaturateOnIntegerOverflow=on
  Demux : Demux  Outputs=4  BusSelectionMode=off
  Memory : Memory  X0=ess_init_soc  InheritSampleTime=off
      settings: RTWStateStorageClass=Auto
  Memory1 : Memory  X0=0  InheritSampleTime=off
      settings: RTWStateStorageClass=Auto
  Memory2 : Memory  X0=0  InheritSampleTime=off
      settings: RTWStateStorageClass=Auto
  Product : Product  Inputs=*/  Multiplication=Element-wise(.*)  SaturateOnIntegerOverflow=on
  To Workspace1 : ToWorkspace  VariableName=ess_current  SampleTime=-1  SaveFormat=Array
  To Workspace2 : ToWorkspace  VariableName=ess_volts  SampleTime=-1  SaveFormat=Array
  To Workspace3 : ToWorkspace  VariableName=ess_max_chg_pwr  SampleTime=-1  SaveFormat=Array
  To Workspace4 : ToWorkspace  VariableName=ess_soc_hist  SampleTime=-1  SaveFormat=Array
  To Workspace5 : ToWorkspace  VariableName=ess_pwr_out_a  SampleTime=-1  SaveFormat=Array
  To Workspace6 : ToWorkspace  VariableName=ess_current_psc  SampleTime=-1  SaveFormat=Array
  psc passive sign convention : Gain  Gain=-1  Multiplication=Element-wise(K.*u)  SaturateOnIntegerOverflow=on
  tag scope: SOC=global, bus_voltage=global, ess_max_chg_pwr=global, ess_pwr_out_a=global
  wires:
  Memory/1 -> [SOC]
  Demux/3 -> To Workspace4/1, Memory/1
  In1/1 -> Demux/1
  Demux/1 -> Advisor sign convention1/1
  Demux/2 -> Memory2/1, Product/2, To Workspace2/1
  Product/1 -> To Workspace1/1, psc passive sign convention/1
  Demux/4 -> Memory1/1, To Workspace3/1
  Memory1/1 -> [ess_max_chg_pwr]
  Memory2/1 -> [bus_voltage]
  psc passive sign convention/1 -> To Workspace6/1
  Advisor sign convention1/1 -> Product/1, To Workspace5/1, [ess_pwr_out_a]

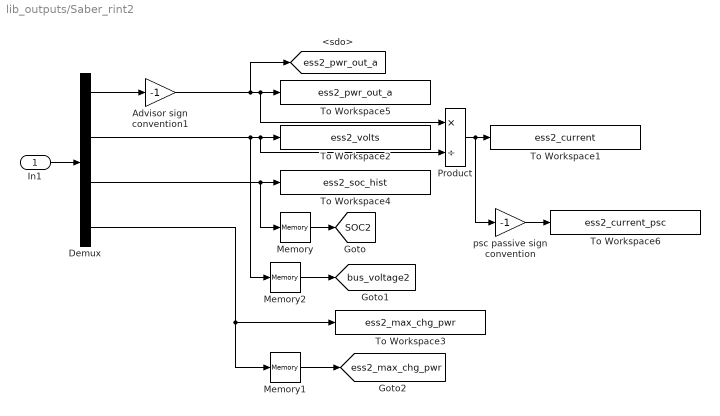
== system lib_outputs/Saber_rint2 ==
  In1 : Inport  Port=1  LatchInput=off
  Advisor sign convention1 : Gain  Gain=-1  Multiplication=Element-wise(K.*u)  SaturateOnIntegerOverflow=on
  Demux : Demux  Outputs=4  BusSelectionMode=off
  Memory : Memory  X0=ess2_init_soc  InheritSampleTime=off
      settings: RTWStateStorageClass=Auto
  Memory1 : Memory  X0=0  InheritSampleTime=off
      settings: RTWStateStorageClass=Auto
  Memory2 : Memory  X0=0  InheritSampleTime=off
      settings: RTWStateStorageClass=Auto
  Product : Product  Inputs=*/  Multiplication=Element-wise(.*)  SaturateOnIntegerOverflow=on
  To Workspace1 : ToWorkspace  VariableName=ess2_current  SampleTime=-1  SaveFormat=Array
  To Workspace2 : ToWorkspace  VariableName=ess2_volts  SampleTime=-1  SaveFormat=Array
  To Workspace3 : ToWorkspace  VariableName=ess2_max_chg_pwr  SampleTime=-1  SaveFormat=Array
  To Workspace4 : ToWorkspace  VariableName=ess2_soc_hist  SampleTime=-1  SaveFormat=Array
  To Workspace5 : ToWorkspace  VariableName=ess2_pwr_out_a  SampleTime=-1  SaveFormat=Array
  To Workspace6 : ToWorkspace  VariableName=ess2_current_psc  SampleTime=-1  SaveFormat=Array
  psc passive sign convention : Gain  Gain=-1  Multiplication=Element-wise(K.*u)  SaturateOnIntegerOverflow=on
  tag scope: SOC2=global, bus_voltage2=global, ess2_max_chg_pwr=global, ess2_pwr_out_a=global
  wires:
  Memory2/1 -> [bus_voltage2]
  Memory1/1 -> [ess2_max_chg_pwr]
  Demux/4 -> To Workspace3/1, Memory1/1
  Product/1 -> To Workspace1/1, psc passive sign convention/1
  Demux/2 -> To Workspace2/1, Product/2, Memory2/1
  Demux/1 -> Advisor sign convention1/1
  In1/1 -> Demux/1
  Demux/3 -> Memory/1, To Workspace4/1
  Memory/1 -> [SOC2]
  psc passive sign convention/1 -> To Workspace6/1
  Advisor sign convention1/1 -> To Workspace5/1, Product/1, [ess2_pwr_out_a]

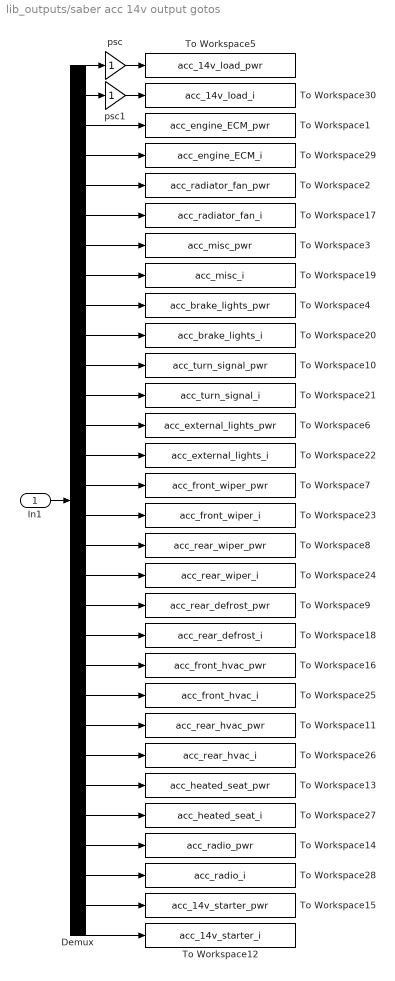
== system lib_outputs/saber acc 14v output gotos ==
  In1 : Inport  Port=1  LatchInput=off
  Demux : Demux  Outputs=30  BusSelectionMode=off
  To Workspace1 : ToWorkspace  VariableName=acc_engine_ECM_pwr  SampleTime=-1  SaveFormat=Array
  To Workspace10 : ToWorkspace  VariableName=acc_turn_signal_pwr  SampleTime=-1  SaveFormat=Array
  To Workspace11 : ToWorkspace  VariableName=acc_rear_hvac_pwr  SampleTime=-1  SaveFormat=Array
  To Workspace12 : ToWorkspace  VariableName=acc_14v_starter_i  SampleTime=-1  SaveFormat=Array
  To Workspace13 : ToWorkspace  VariableName=acc_heated_seat_pwr  SampleTime=-1  SaveFormat=Array
  To Workspace14 : ToWorkspace  VariableName=acc_radio_pwr  SampleTime=-1  SaveFormat=Array
  To Workspace15 : ToWorkspace  VariableName=acc_14v_starter_pwr  SampleTime=-1  SaveFormat=Array
  To Workspace16 : ToWorkspace  VariableName=acc_front_hvac_pwr  SampleTime=-1  SaveFormat=Array
  To Workspace17 : ToWorkspace  VariableName=acc_radiator_fan_i  SampleTime=-1  SaveFormat=Array
  To Workspace18 : ToWorkspace  VariableName=acc_rear_defrost_i  SampleTime=-1  SaveFormat=Array
  To Workspace19 : ToWorkspace  VariableName=acc_misc_i  SampleTime=-1  SaveFormat=Array
  To Workspace2 : ToWorkspace  VariableName=acc_radiator_fan_pwr  SampleTime=-1  SaveFormat=Array
  To Workspace20 : ToWorkspace  VariableName=acc_brake_lights_i  SampleTime=-1  SaveFormat=Array
  To Workspace21 : ToWorkspace  VariableName=acc_turn_signal_i  SampleTime=-1  SaveFormat=Array
  To Workspace22 : ToWorkspace  VariableName=acc_external_lights_i  SampleTime=-1  SaveFormat=Array
  To Workspace23 : ToWorkspace  VariableName=acc_front_wiper_i  SampleTime=-1  SaveFormat=Array
  To Workspace24 : ToWorkspace  VariableName=acc_rear_wiper_i  SampleTime=-1  SaveFormat=Array
  To Workspace25 : ToWorkspace  VariableName=acc_front_hvac_i  SampleTime=-1  SaveFormat=Array
  To Workspace26 : ToWorkspace  VariableName=acc_rear_hvac_i  SampleTime=-1  SaveFormat=Array
  To Workspace27 : ToWorkspace  VariableName=acc_heated_seat_i  SampleTime=-1  SaveFormat=Array
  To Workspace28 : ToWorkspace  VariableName=acc_radio_i  SampleTime=-1  SaveFormat=Array
  To Workspace29 : ToWorkspace  VariableName=acc_engine_ECM_i  SampleTime=-1  SaveFormat=Array
  To Workspace3 : ToWorkspace  VariableName=acc_misc_pwr  SampleTime=-1  SaveFormat=Array
  To Workspace30 : ToWorkspace  VariableName=acc_14v_load_i  SampleTime=-1  SaveFormat=Array
  To Workspace4 : ToWorkspace  VariableName=acc_brake_lights_pwr  SampleTime=-1  SaveFormat=Array
  To Workspace5 : ToWorkspace  VariableName=acc_14v_load_pwr  SampleTime=-1  SaveFormat=Array
  To Workspace6 : ToWorkspace  VariableName=acc_external_lights_pwr  SampleTime=-1  SaveFormat=Array
  To Workspace7 : ToWorkspace  VariableName=acc_front_wiper_pwr  SampleTime=-1  SaveFormat=Array
  To Workspace8 : ToWorkspace  VariableName=acc_rear_wiper_pwr  SampleTime=-1  SaveFormat=Array
  To Workspace9 : ToWorkspace  VariableName=acc_rear_defrost_pwr  SampleTime=-1  SaveFormat=Array
  psc : Gain  Gain=1  Multiplication=Element-wise(K.*u)  SaturateOnIntegerOverflow=on
  psc1 : Gain  Gain=1  Multiplication=Element-wise(K.*u)  SaturateOnIntegerOverflow=on
  wires:
  Demux/7 -> To Workspace3/1
  Demux/3 -> To Workspace1/1
  Demux/9 -> To Workspace4/1
  Demux/1 -> psc/1
  Demux/5 -> To Workspace2/1
  Demux/17 -> To Workspace8/1
  Demux/13 -> To Workspace6/1
  Demux/19 -> To Workspace9/1
  Demux/11 -> To Workspace10/1
  Demux/15 -> To Workspace7/1
  Demux/27 -> To Workspace14/1
  Demux/23 -> To Workspace11/1
  Demux/21 -> To Workspace16/1
  Demux/25 -> To Workspace13/1
  Demux/6 -> To Workspace17/1
  In1/1 -> Demux/1
  Demux/20 -> To Workspace18/1
  Demux/22 -> To Workspace25/1
  Demux/24 -> To Workspace26/1
  Demux/26 -> To Workspace27/1
  Demux/28 -> To Workspace28/1
  Demux/8 -> To Workspace19/1
  Demux/10 -> To Workspace20/1
  Demux/12 -> To Workspace21/1
  Demux/14 -> To Workspace22/1
  Demux/16 -> To Workspace23/1
  Demux/18 -> To Workspace24/1
  Demux/4 -> To Workspace29/1
  Demux/29 -> To Workspace15/1
  Demux/30 -> To Workspace12/1
  Demux/2 -> psc1/1
  psc/1 -> To Workspace5/1
  psc1/1 -> To Workspace30/1

== system lib_outputs/saber acc HiV output gotos ==
  note: Note: psc : passive sign convention
  In1 : Inport  Port=1  LatchInput=off
  Demux : Demux  Outputs=12  BusSelectionMode=off
  To Workspace1 : ToWorkspace  VariableName=acc_HiV_load_pwr  SampleTime=-1  SaveFormat=Array
  To Workspace15 : ToWorkspace  VariableName=acc_speed_load_pwr  SampleTime=-1  SaveFormat=Array
  To Workspace17 : ToWorkspace  VariableName=acc_HiV_pwr_load_1_pwr  SampleTime=-1  SaveFormat=Array
  To Workspace18 : ToWorkspace  VariableName=acc_HiV_pwr_load_2_pwr  SampleTime=-1  SaveFormat=Array
  To Workspace19 : ToWorkspace  VariableName=acc_HiV_pwr_load_3_pwr  SampleTime=-1  SaveFormat=Array
  To Workspace2 : ToWorkspace  VariableName=acc_HiV_starter_pwr  SampleTime=-1  SaveFormat=Array
  To Workspace20 : ToWorkspace  VariableName=acc_HiV_starter_i  SampleTime=-1  SaveFormat=Array
  To Workspace3 : ToWorkspace  VariableName=acc_speed_load_i  SampleTime=-1  SaveFormat=Array
  To Workspace4 : ToWorkspace  VariableName=acc_HiV_pwr_load_1_i  SampleTime=-1  SaveFormat=Array
  To Workspace5 : ToWorkspace  VariableName=acc_HiV_pwr_load_2_i  SampleTime=-1  SaveFormat=Array
  To Workspace6 : ToWorkspace  VariableName=acc_HiV_pwr_load_3_i  SampleTime=-1  SaveFormat=Array
  To Workspace7 : ToWorkspace  VariableName=acc_HiV_load_i  SampleTime=-1  SaveFormat=Array
  psc : Gain  Gain=1  Multiplication=Element-wise(K.*u)  SaturateOnIntegerOverflow=on
  psc1 : Gain  Gain=1  Multiplication=Element-wise(K.*u)  SaturateOnIntegerOverflow=on
  wires:
  Demux/7 -> To Workspace18/1
  Demux/5 -> To Workspace17/1
  Demux/9 -> To Workspace19/1
  Demux/3 -> To Workspace15/1
  In1/1 -> Demux/1
  Demux/1 -> psc1/1
  Demux/4 -> To Workspace3/1
  Demux/6 -> To Workspace4/1
  Demux/8 -> To Workspace5/1
  Demux/10 -> To Workspace6/1
  Demux/11 -> To Workspace2/1
  Demux/12 -> To Workspace20/1
  Demux/2 -> psc/1
  psc/1 -> To Workspace7/1
  psc1/1 -> To Workspace1/1

== system lib_outputs/saber acc additional outputs ==
  In1 : Inport  Port=1  LatchInput=off
  Demux : Demux  Outputs=2  BusSelectionMode=off
  To Workspace1 : ToWorkspace  VariableName=acc_elec_i_a  SampleTime=-1  SaveFormat=Array
  To Workspace5 : ToWorkspace  VariableName=acc_elec_pwr_a  SampleTime=-1  SaveFormat=Array
  wires:
  In1/1 -> Demux/1
  Demux/1 -> To Workspace5/1
  Demux/2 -> To Workspace1/1

== system lib_outputs/saber dcdc output gotos ==
  In1 : Inport  Port=1  LatchInput=off
  Demux : Demux  Outputs=2  BusSelectionMode=off
  To Workspace5 : ToWorkspace  VariableName=ess2_dcdc_i_out  SampleTime=-1  SaveFormat=Array
  To Workspace6 : ToWorkspace  VariableName=ess2_dcdc_i_in  SampleTime=-1  SaveFormat=Array
  wires:
  Demux/1 -> To Workspace6/1
  In1/1 -> Demux/1
  Demux/2 -> To Workspace5/1

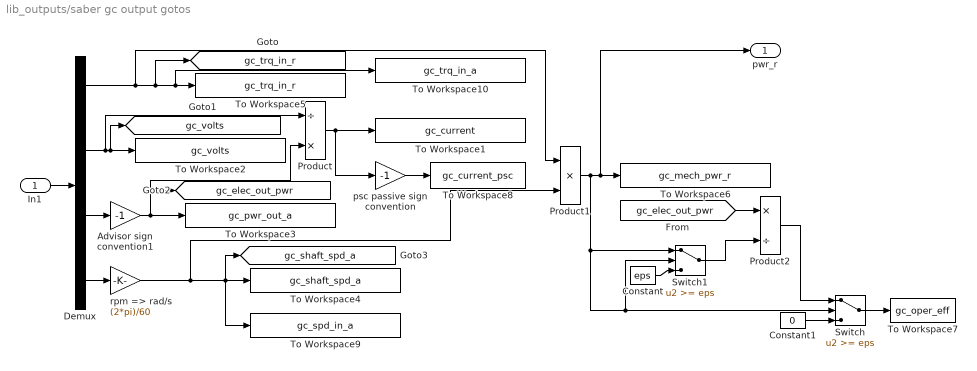
== system lib_outputs/saber gc output gotos ==
  In1 : Inport  Port=1  LatchInput=off
  Advisor sign convention1 : Gain  Gain=-1  Multiplication=Element-wise(K.*u)  SaturateOnIntegerOverflow=on
  Constant : Constant  Value=eps
  Constant1 : Constant  Value=0
  Demux : Demux  Outputs=4  BusSelectionMode=off
  Product : Product  Inputs=/*  Multiplication=Element-wise(.*)  SaturateOnIntegerOverflow=on
  Product1 : Product  Inputs=**  Multiplication=Element-wise(.*)  SaturateOnIntegerOverflow=on
  Product2 : Product  Inputs=*/  Multiplication=Element-wise(.*)  SaturateOnIntegerOverflow=on
  Switch : Switch  Threshold=eps
  Switch1 : Switch  Threshold=eps
  To Workspace1 : ToWorkspace  VariableName=gc_current  SampleTime=-1  SaveFormat=Array
  To Workspace10 : ToWorkspace  VariableName=gc_trq_in_a  SampleTime=-1  SaveFormat=Array
  To Workspace2 : ToWorkspace  VariableName=gc_volts  SampleTime=-1  SaveFormat=Array
  To Workspace3 : ToWorkspace  VariableName=gc_pwr_out_a  SampleTime=-1  SaveFormat=Array
  To Workspace4 : ToWorkspace  VariableName=gc_shaft_spd_a  SampleTime=-1  SaveFormat=Array
  To Workspace5 : ToWorkspace  VariableName=gc_trq_in_r  SampleTime=-1  SaveFormat=Array
  To Workspace6 : ToWorkspace  VariableName=gc_mech_pwr_r  SampleTime=-1  SaveFormat=Array
  To Workspace7 : ToWorkspace  VariableName=gc_oper_eff  SampleTime=-1  SaveFormat=Array
  To Workspace8 : ToWorkspace  VariableName=gc_current_psc  SampleTime=-1  SaveFormat=Array
  To Workspace9 : ToWorkspace  VariableName=gc_spd_in_a  SampleTime=-1  SaveFormat=Array
  psc passive sign convention : Gain  Gain=-1  Multiplication=Element-wise(K.*u)  SaturateOnIntegerOverflow=on
  rpm => rad/s : Gain  Gain=(2*pi)/60  Multiplication=Element-wise(K.*u)  SaturateOnIntegerOverflow=on
  pwr_r : Outport  Port=1
  tag scope: gc_elec_out_pwr=global, gc_shaft_spd_a=global, gc_trq_in_r=global, gc_volts=global
  wires:
  Demux/2 -> Product/1, To Workspace2/1, [gc_volts]
  Demux/1 -> Product1/1, [gc_trq_in_r], To Workspace5/1, To Workspace10/1
  In1/1 -> Demux/1
  Demux/4 -> rpm => rad/s/1
  Demux/3 -> Advisor sign convention1/1
  Product/1 -> To Workspace1/1, psc passive sign convention/1
  Product1/1 -> To Workspace6/1, pwr_r/1, Switch/2, Switch1/2, Switch1/1
  rpm => rad/s/1 -> Product1/2, To Workspace4/1, [gc_shaft_spd_a], To Workspace9/1
  Switch/1 -> To Workspace7/1
  Product2/1 -> Switch/1
  [gc_elec_out_pwr] -> Product2/1
  Switch1/1 -> Product2/2
  Constant/1 -> Switch1/3
  Constant1/1 -> Switch/3
  psc passive sign convention/1 -> To Workspace8/1
  Advisor sign convention1/1 -> Product/2, [gc_elec_out_pwr], To Workspace3/1

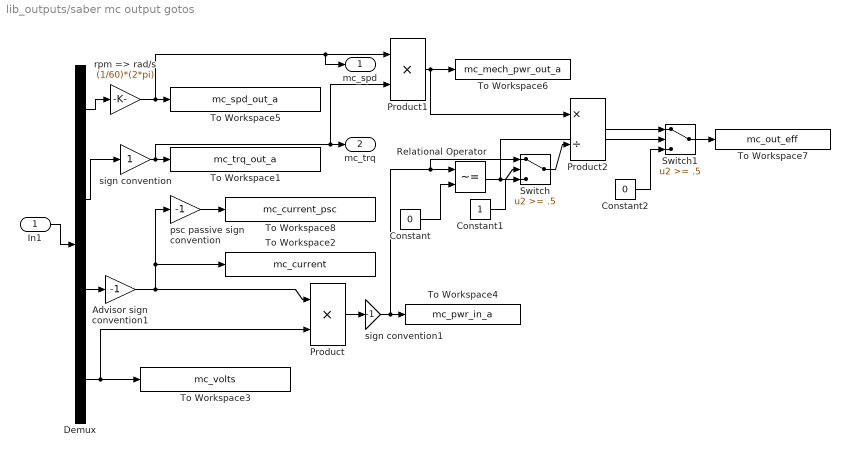
== system lib_outputs/saber mc output gotos ==
  In1 : Inport  Port=1  LatchInput=off
  Advisor sign convention1 : Gain  Gain=-1  Multiplication=Element-wise(K.*u)  SaturateOnIntegerOverflow=on
  Constant : Constant  Value=0
  Constant1 : Constant  Value=1
  Constant2 : Constant  Value=0
  Demux : Demux  Outputs=4  BusSelectionMode=off
  Product : Product  Inputs=**  Multiplication=Element-wise(.*)  SaturateOnIntegerOverflow=on
  Product1 : Product  Inputs=**  Multiplication=Element-wise(.*)  SaturateOnIntegerOverflow=on
  Product2 : Product  Inputs=*/  Multiplication=Element-wise(.*)  SaturateOnIntegerOverflow=on
  Relational Operator : RelationalOperator  Operator=~=
  Switch : Switch  Threshold=.5
  Switch1 : Switch  Threshold=.5
  To Workspace1 : ToWorkspace  VariableName=mc_trq_out_a  SampleTime=-1  SaveFormat=Array
  To Workspace2 : ToWorkspace  VariableName=mc_current  SampleTime=-1  SaveFormat=Array
  To Workspace3 : ToWorkspace  VariableName=mc_volts  SampleTime=-1  SaveFormat=Array
  To Workspace4 : ToWorkspace  VariableName=mc_pwr_in_a  SampleTime=-1  SaveFormat=Array
  To Workspace5 : ToWorkspace  VariableName=mc_spd_out_a  SampleTime=-1  SaveFormat=Array
  To Workspace6 : ToWorkspace  VariableName=mc_mech_pwr_out_a  SampleTime=-1  SaveFormat=Array
  To Workspace7 : ToWorkspace  VariableName=mc_out_eff  SampleTime=-1  SaveFormat=Array
  To Workspace8 : ToWorkspace  VariableName=mc_current_psc  SampleTime=-1  SaveFormat=Array
  psc passive sign convention : Gain  Gain=-1  Multiplication=Element-wise(K.*u)  SaturateOnIntegerOverflow=on
  rpm => rad/s : Gain  Gain=(1/60)*(2*pi)  Multiplication=Element-wise(K.*u)  SaturateOnIntegerOverflow=on
  sign convention : Gain  Gain=1  Multiplication=Element-wise(K.*u)  SaturateOnIntegerOverflow=on
  sign convention1 : Gain  Gain=-1  Multiplication=Element-wise(K.*u)  SaturateOnIntegerOverflow=on
  mc_spd : Outport  Port=1
  mc_trq : Outport  Port=2
  wires:
  Demux/4 -> To Workspace3/1, Product/2
  Demux/2 -> sign convention/1
  Product/1 -> sign convention1/1
  In1/1 -> Demux/1
  Demux/1 -> rpm => rad/s/1
  Demux/3 -> Advisor sign convention1/1
  sign convention/1 -> To Workspace1/1, mc_trq/1, Product1/2
  rpm => rad/s/1 -> To Workspace5/1, mc_spd/1, Product1/1
  Product1/1 -> To Workspace6/1, Product2/1
  Relational Operator/1 -> Switch/2, Switch1/2
  Constant/1 -> Relational Operator/2
  Constant1/1 -> Switch/3
  Switch/1 -> Product2/2
  Switch1/1 -> To Workspace7/1
  Product2/1 -> Switch1/1
  Constant2/1 -> Switch1/3
  sign convention1/1 -> To Workspace4/1, Relational Operator/1, Switch/1
  psc passive sign convention/1 -> To Workspace8/1
  Advisor sign convention1/1 -> Product/1, To Workspace2/1, psc passive sign convention/1
